simulink subsystem "PreCharge"  (R2023b)
settings: Solver=VariableStepAuto  StartTime=0.0  StopTime=10.0  RelTol=1e-3
libraries: simrfV2elements x2, simrfV2util1 x2, simrfV2_lib x1
settings Model: Creator=heyka  LastModifiedBy=diego
settings DebuggingCC: UnconnectedInputMsg=warning  UnconnectedOutputMsg=warning  UnconnectedLineMsg=warning
settings ModelReferenceCC: EnableRefExpFcnMdlSchedulingChecks=on
settings RTWCC: DLArmComputeVersion=19.05

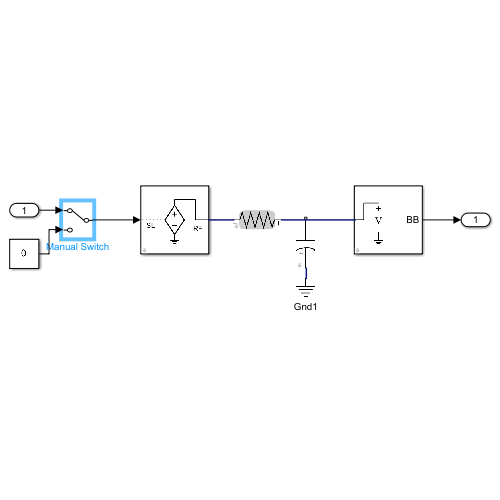
[thumbnail: Simulink's stored preview of the top-level diagram]
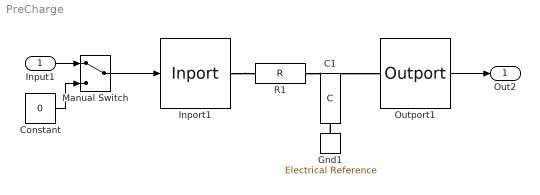
== system PreCharge ==
  Input1 : Inport
  C1 : simrfV2elements/C  classname=capacitor  Capacitance=500 uF
  Constant : Constant  Value=0
  Gnd1 : simrfV2_lib/Elements/Electrical Reference
      settings: LibrarySourceBlock=simrfV2elements/Gnd  InternalSimscapePortConfiguration="{\"Bottom\":[],\"Left\":[{\"id\":\"V\",\"label\":\"\",\"type\":\"foundation.rf.circuitenvelope\"}],\"Right\":[],\"Top\":[]}"
  Inport1 : simrfV2util1/Inport  SimulinkInputSignalType=Ideal voltage  CarrierFreq=0 Hz  ZS=0  UseSqWave=off  NumCoeff=10  Bias=0  DutyCyc=50  InternalGrounding=on
  Manual Switch : ManualSwitch
  Outport1 : simrfV2util1/Outport  SensorType=Ideal voltage  OutputFormat=Complex Baseband  CarrierFreq=0 Hz  ZL=Inf  InternalGrounding=on  StepSize=1e-6 s  AutoStep=on  HalfPolyphaseLength=12
  R1 : simrfV2elements/R  classname=resistor  Resistance=560 Ohm  AddNoise=on
  Out2 : Outport
  wires:
  Manual Switch/1 -> Inport1/1
  Constant/1 -> Manual Switch/2
  Input1/1 -> Manual Switch/1
  Outport1/1 -> Out2/1
  connections:
  Inport1/RConn1 -- R1/LConn1
  R1/RConn1 -- Outport1/LConn1
  Gnd1/LConn1 -- C1/RConn1
